simulink model "main_mmp_frac"  (R2024a)
settings: Solver=VariableStepAuto  StartTime=0.0  StopTime=Tsim  FixedStep=simStepSize  RelTol=1e-3
undefined symbols (not defined in the file): A_amp, B_para, f_hz, ForceDist, L_t, mmp_fir_coeff, mmp_iir_coeff, p_off, Ps_sys, Pz_sys, Qcvx_sim, SensorNoise, T_cs, T_fs, T_ss
libraries: cstblocks x2
settings Model: Creator=tomli  LastModifiedBy=tpjch
settings RTWCC: GPUComputeCapability=3.5

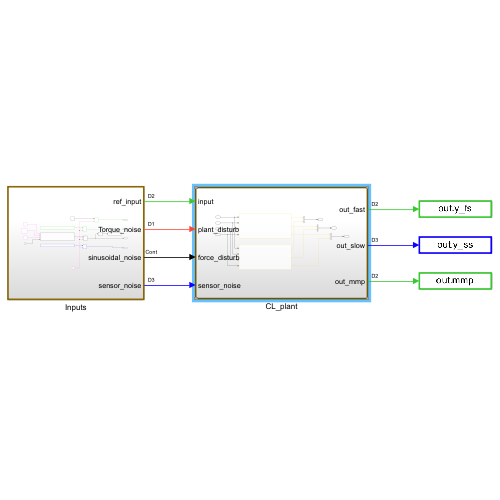
[thumbnail: Simulink's stored preview of the top-level diagram]
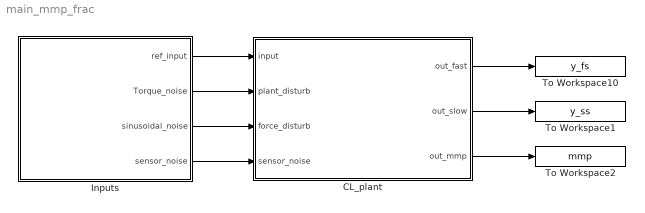
== system main_mmp_frac ==
  CL_plant : Subsystem
  Inputs : Subsystem
  To Workspace1 : ToWorkspace  VariableName=y_ss  SaveFormat=Structure With Time  SampleTime=-1
  To Workspace10 : ToWorkspace  VariableName=y_fs  SaveFormat=Structure With Time  SampleTime=-1
  To Workspace2 : ToWorkspace  VariableName=mmp  SaveFormat=Structure With Time  SampleTime=-1
  wires:
  Inputs/1(ref_input) -> CL_plant/1(input)
  Inputs/2(Torque_noise) -> CL_plant/2(plant_disturb)
  Inputs/3(sinusoidal_noise) -> CL_plant/3(force_disturb)
  Inputs/4(sensor_noise) -> CL_plant/4(sensor_noise)
  CL_plant/1(out_fast) -> To Workspace10/1
  CL_plant/2(out_slow) -> To Workspace1/1
  CL_plant/3(out_mmp) -> To Workspace2/1

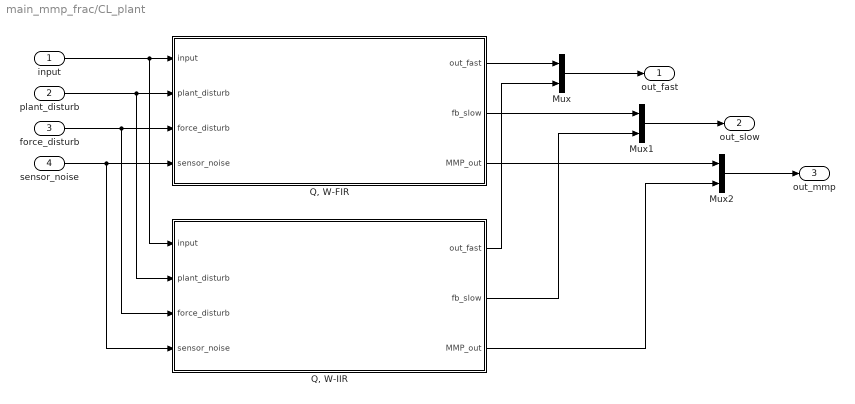
== system main_mmp_frac/CL_plant ==
  input : Inport
  plant_disturb : Inport  Port=2
  force_disturb : Inport  Port=3
  sensor_noise : Inport  Port=4
  Mux : Mux  Inputs=2
  Mux1 : Mux  Inputs=2
  Mux2 : Mux  Inputs=2
  "Q, W-FIR" : Subsystem
  "Q, W-IIR" : Subsystem
  out_fast : Outport
  out_slow : Outport  Port=2
  out_mmp : Outport  Port=3
  wires:
  sensor_noise/1 -> "Q, W-IIR"/4(sensor_noise), "Q, W-FIR"/4(sensor_noise)
  "Q, W-FIR"/2(fb_slow) -> Mux1/1
  Mux1/1 -> out_slow/1
  "Q, W-IIR"/1(out_fast) -> Mux/2
  plant_disturb/1 -> "Q, W-IIR"/2(plant_disturb), "Q, W-FIR"/2(plant_disturb)
  force_disturb/1 -> "Q, W-IIR"/3(force_disturb), "Q, W-FIR"/3(force_disturb)
  "Q, W-FIR"/1(out_fast) -> Mux/1
  input/1 -> "Q, W-IIR"/1(input), "Q, W-FIR"/1(input)
  "Q, W-FIR"/3(MMP_out) -> Mux2/1
  Mux/1 -> out_fast/1
  Mux2/1 -> out_mmp/1
  "Q, W-IIR"/3(MMP_out) -> Mux2/2
  "Q, W-IIR"/2(fb_slow) -> Mux1/2

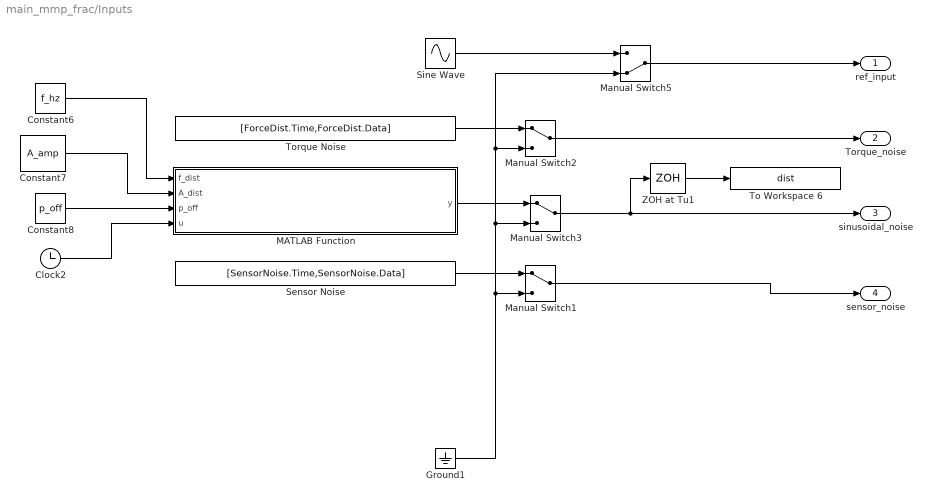
== system main_mmp_frac/Inputs ==
  Clock2 : Clock
  Constant6 : Constant  Value=f_hz
  Constant7 : Constant  Value=A_amp
  Constant8 : Constant  Value=p_off
  Ground1 : Ground
  MATLAB Function : MATLAB Function  TreatAsAtomicUnit=on
  Manual Switch1 : ManualSwitch
  Manual Switch2 : ManualSwitch
  Manual Switch3 : ManualSwitch
  Manual Switch5 : ManualSwitch  CurrentSetting=0
  Sensor Noise : FromWorkspace  VariableName=[SensorNoise.Time,SensorNoise.Data]  SampleTime=SensorNoise.Ts  Interpolate=off  ZeroCross=off  OutputAfterFinalValue=Setting to zero
  Sine Wave : Sin  SampleTime=T_fs
  To Workspace 6 : ToWorkspace  VariableName=dist  SaveFormat=Structure With Time  SampleTime=T_fs
      settings: MaxDataPoints=Inf
  Torque Noise : FromWorkspace  VariableName=[ForceDist.Time,ForceDist.Data]  SampleTime=ForceDist.Ts  Interpolate=off  ZeroCross=off  OutputAfterFinalValue=Setting to zero
  ZOH at Tu1 : ZeroOrderHold  SampleTime=T_fs
  ref_input : Outport
  Torque_noise : Outport  Port=2
  sinusoidal_noise : Outport  Port=3
  sensor_noise : Outport  Port=4
  wires:
  Torque Noise/1 -> Manual Switch2/1
  Constant7/1 -> MATLAB Function/2(A_dist)
  Manual Switch1/1 -> sensor_noise/1
  Constant8/1 -> MATLAB Function/3(p_off)
  MATLAB Function/1(y) -> Manual Switch3/1
  Clock2/1 -> MATLAB Function/4(u)
  Constant6/1 -> MATLAB Function/1(f_dist)
  ZOH at Tu1/1 -> To Workspace 6/1
  Manual Switch3/1 -> sinusoidal_noise/1, ZOH at Tu1/1
  Sensor Noise/1 -> Manual Switch1/1
  Manual Switch2/1 -> Torque_noise/1
  Manual Switch5/1 -> ref_input/1
  Sine Wave/1 -> Manual Switch5/1
  Ground1/1 -> Manual Switch5/2, Manual Switch2/2, Manual Switch3/2, Manual Switch1/2

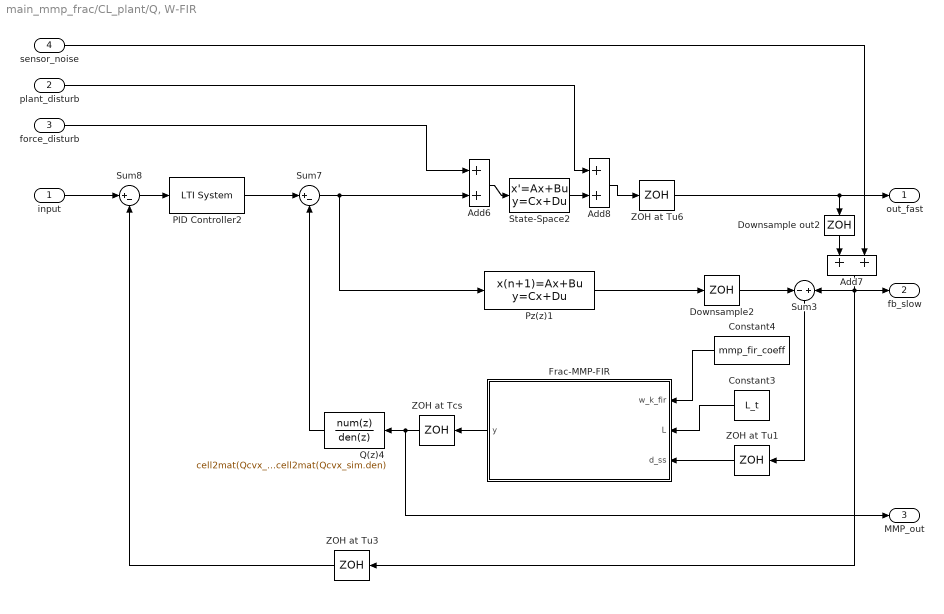
== system main_mmp_frac/CL_plant/Q, W-FIR ==
  input : Inport
  plant_disturb : Inport  Port=2
  force_disturb : Inport  Port=3
  sensor_noise : Inport  Port=4
  Add6 : Sum
  Add7 : Sum
  Add8 : Sum
  Constant3 : Constant  Value=L_t
  Constant4 : Constant  Value=mmp_fir_coeff
  Downsample out2 : ZeroOrderHold  SampleTime=T_ss
  Downsample2 : ZeroOrderHold  SampleTime=T_ss
  Frac-MMP-FIR : Subsystem
  PID Controller2 : cstblocks/LTI System  sys=Cz  IC=[]  PadeOrder=0
  Pz(z)1 : DiscreteStateSpace  A=Pz_sys.A  B=Pz_sys.B  C=Pz_sys.C  D=Pz_sys.D  SampleTime=T_fs
  Q(z)4 : DiscreteTransferFcn  Numerator=cell2mat(Qcvx_sim.num)  Denominator=cell2mat(Qcvx_sim.den)
  State-Space2 : StateSpace  A=Ps_sys.A  B=Ps_sys.B  C=Ps_sys.C  D=Ps_sys.D  InitialCondition=0
  Sum3 : Sum  Inputs=-|+
  Sum7 : Sum  Inputs=|+-
  Sum8 : Sum  Inputs=|+-
  ZOH at Tcs : ZeroOrderHold  SampleTime=T_fs
  ZOH at Tu1 : ZeroOrderHold  SampleTime=T_cs
  ZOH at Tu3 : ZeroOrderHold  SampleTime=T_fs
  ZOH at Tu6 : ZeroOrderHold  SampleTime=T_fs
  out_fast : Outport
  fb_slow : Outport  Port=2
  MMP_out : Outport  Port=3
  wires:
  Q(z)4/1 -> Sum7/2
  ZOH at Tu1/1 -> Frac-MMP-FIR/3(d_ss)
  Frac-MMP-FIR/1(y) -> ZOH at Tcs/1
  Constant4/1 -> Frac-MMP-FIR/1(w_k_fir)
  Constant3/1 -> Frac-MMP-FIR/2(L)
  Sum3/1 -> ZOH at Tu1/1
  Downsample2/1 -> Sum3/1
  ZOH at Tcs/1 -> Q(z)4/1, MMP_out/1
  force_disturb/1 -> Add6/1
  Add6/1 -> State-Space2/1
  ZOH at Tu6/1 -> out_fast/1, Downsample out2/1
  Add8/1 -> ZOH at Tu6/1
  plant_disturb/1 -> Add8/1
  Downsample out2/1 -> Add7/1
  Pz(z)1/1 -> Downsample2/1
  State-Space2/1 -> Add8/2
  ZOH at Tu3/1 -> Sum8/2
  Sum7/1 -> Add6/2, Pz(z)1/1
  sensor_noise/1 -> Add7/2
  Sum8/1 -> PID Controller2/1
  input/1 -> Sum8/1
  PID Controller2/1 -> Sum7/1
  Add7/1 -> ZOH at Tu3/1, fb_slow/1, Sum3/2

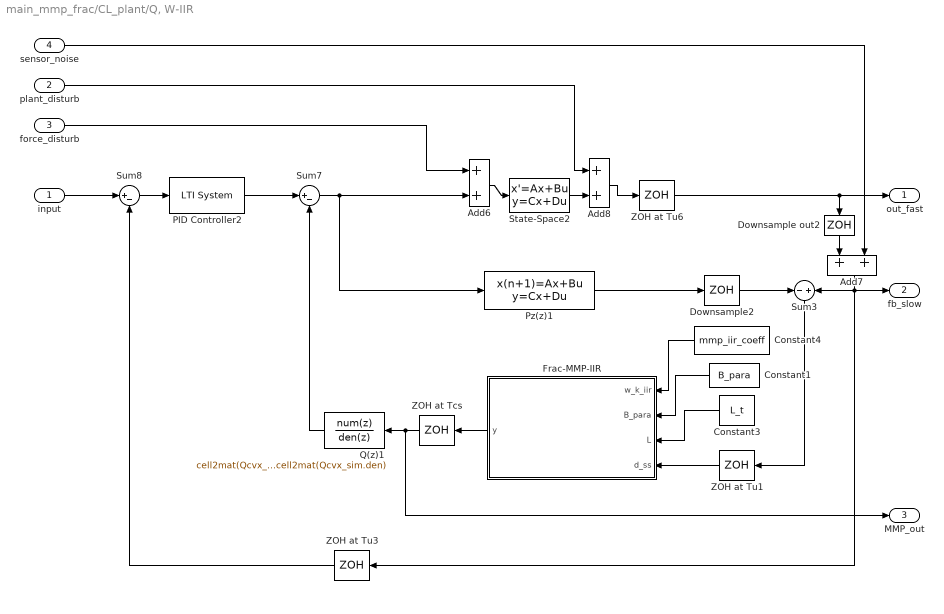
== system main_mmp_frac/CL_plant/Q, W-IIR ==
  input : Inport
  plant_disturb : Inport  Port=2
  force_disturb : Inport  Port=3
  sensor_noise : Inport  Port=4
  Add6 : Sum
  Add7 : Sum
  Add8 : Sum
  Constant1 : Constant  Value=B_para
  Constant3 : Constant  Value=L_t
  Constant4 : Constant  Value=mmp_iir_coeff
  Downsample out2 : ZeroOrderHold  SampleTime=T_ss
  Downsample2 : ZeroOrderHold  SampleTime=T_ss
  Frac-MMP-IIR : Subsystem
  PID Controller2 : cstblocks/LTI System  sys=Cz  IC=[]  PadeOrder=0
  Pz(z)1 : DiscreteStateSpace  A=Pz_sys.A  B=Pz_sys.B  C=Pz_sys.C  D=Pz_sys.D  SampleTime=T_fs
  Q(z)1 : DiscreteTransferFcn  Numerator=cell2mat(Qcvx_sim.num)  Denominator=cell2mat(Qcvx_sim.den)
  State-Space2 : StateSpace  A=Ps_sys.A  B=Ps_sys.B  C=Ps_sys.C  D=Ps_sys.D  InitialCondition=0
  Sum3 : Sum  Inputs=-|+
  Sum7 : Sum  Inputs=|+-
  Sum8 : Sum  Inputs=|+-
  ZOH at Tcs : ZeroOrderHold  SampleTime=T_fs
  ZOH at Tu1 : ZeroOrderHold  SampleTime=T_cs
  ZOH at Tu3 : ZeroOrderHold  SampleTime=T_fs
  ZOH at Tu6 : ZeroOrderHold  SampleTime=T_fs
  out_fast : Outport
  fb_slow : Outport  Port=2
  MMP_out : Outport  Port=3
  wires:
  Add7/1 -> ZOH at Tu3/1, fb_slow/1, Sum3/2
  Sum7/1 -> Add6/2, Pz(z)1/1
  Pz(z)1/1 -> Downsample2/1
  sensor_noise/1 -> Add7/2
  Downsample out2/1 -> Add7/1
  plant_disturb/1 -> Add8/1
  input/1 -> Sum8/1
  Add8/1 -> ZOH at Tu6/1
  Sum8/1 -> PID Controller2/1
  ZOH at Tu3/1 -> Sum8/2
  PID Controller2/1 -> Sum7/1
  Downsample2/1 -> Sum3/1
  force_disturb/1 -> Add6/1
  ZOH at Tcs/1 -> Q(z)1/1, MMP_out/1
  Add6/1 -> State-Space2/1
  Sum3/1 -> ZOH at Tu1/1
  Constant1/1 -> Frac-MMP-IIR/2(B_para)
  Q(z)1/1 -> Sum7/2
  Constant3/1 -> Frac-MMP-IIR/3(L)
  State-Space2/1 -> Add8/2
  Constant4/1 -> Frac-MMP-IIR/1(w_k_iir)
  ZOH at Tu6/1 -> out_fast/1, Downsample out2/1
  ZOH at Tu1/1 -> Frac-MMP-IIR/4(d_ss)
  Frac-MMP-IIR/1(y) -> ZOH at Tcs/1

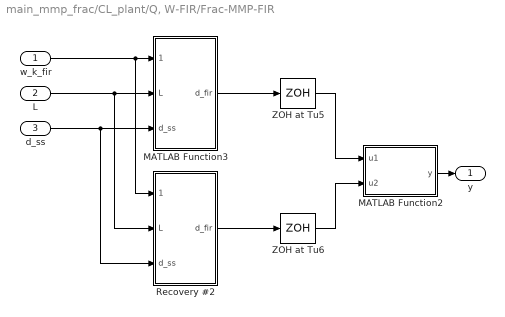
== system main_mmp_frac/CL_plant/Q, W-FIR/Frac-MMP-FIR ==
  w_k_fir : Inport
  L : Inport  Port=2
  d_ss : Inport  Port=3
  MATLAB Function2 : MATLAB Function  TreatAsAtomicUnit=on
  MATLAB Function3 : MATLAB Function  TreatAsAtomicUnit=on  SystemSampleTime=T_cs
  Recovery #2 : MATLAB Function  TreatAsAtomicUnit=on  SystemSampleTime=T_cs
  ZOH at Tu5 : ZeroOrderHold  SampleTime=T_cs
  ZOH at Tu6 : ZeroOrderHold  SampleTime=T_cs
  y : Outport
  wires:
  MATLAB Function2/1(y) -> y/1
  L/1 -> Recovery #2/2(L), MATLAB Function3/2(L)
  w_k_fir/1 -> Recovery #2/1(w_k_fir), MATLAB Function3/1(w_k_fir)
  ZOH at Tu5/1 -> MATLAB Function2/1(u1)
  MATLAB Function3/1(d_fir) -> ZOH at Tu5/1
  Recovery #2/1(d_fir) -> ZOH at Tu6/1
  ZOH at Tu6/1 -> MATLAB Function2/2(u2)
  d_ss/1 -> Recovery #2/3(d_ss), MATLAB Function3/3(d_ss)

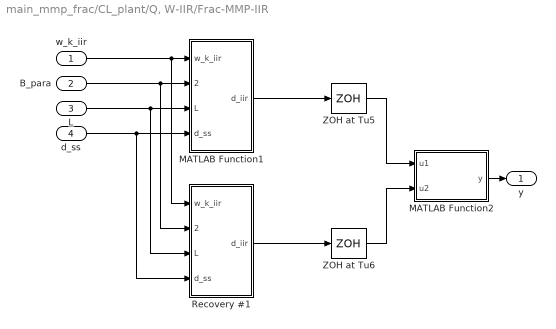
== system main_mmp_frac/CL_plant/Q, W-IIR/Frac-MMP-IIR ==
  w_k_iir : Inport
  B_para : Inport  Port=2
  L : Inport  Port=3
  d_ss : Inport  Port=4
  MATLAB Function1 : MATLAB Function  TreatAsAtomicUnit=on  SystemSampleTime=T_cs
  MATLAB Function2 : MATLAB Function  TreatAsAtomicUnit=on
  Recovery #1 : MATLAB Function  TreatAsAtomicUnit=on  SystemSampleTime=T_cs
  ZOH at Tu5 : ZeroOrderHold  SampleTime=T_cs
  ZOH at Tu6 : ZeroOrderHold  SampleTime=T_cs
  y : Outport
  wires:
  MATLAB Function2/1(y) -> y/1
  L/1 -> Recovery #1/3(L), MATLAB Function1/3(L)
  w_k_iir/1 -> Recovery #1/1(w_k_iir), MATLAB Function1/1(w_k_iir)
  ZOH at Tu5/1 -> MATLAB Function2/1(u1)
  MATLAB Function1/1(d_iir) -> ZOH at Tu5/1
  Recovery #1/1(d_iir) -> ZOH at Tu6/1
  ZOH at Tu6/1 -> MATLAB Function2/2(u2)
  B_para/1 -> Recovery #1/2(B_para), MATLAB Function1/2(B_para)
  d_ss/1 -> Recovery #1/4(d_ss), MATLAB Function1/4(d_ss)

== matlab function main_mmp_frac/Inputs/MATLAB Function ==
  data: f_dist input; A_dist input; p_off input; u input; y output
function y = fcn(f_dist,A_dist,p_off,u)
y = zeros(1,length(u));
for i = 1:length(f_dist)
y = y + A_dist(i)*sin(2*pi*f_dist(i)*u+p_off(i));
end

== matlab function main_mmp_frac/CL_plant/Q, W-IIR/Frac-MMP-IIR/Recovery #1 ==
  settings: updateMethod=DISCRETE
  data: w_k_iir input; B_para input; L input; d_ss input; d_iir output
function d_iir  = fcn(w_k_iir, B_para, L, d_ss)
    % Keeps data of variables
    persistent  n_w phi n_cs n_ss d_buff d_fs_iir max_buffer_size buffer_indices N_L D_L
    % Assigning initial values   
    if isempty(n_w)
        n_w = size(w_k_iir,1); % n_w = 2m disturbances (index starts at 0,1,...,2m-1)
        phi = zeros(1, n_w, 'like', d_ss); % Preallocate phi using the same type as d_ss
        [N_L, D_L] = rat(L);
        n_cs = -N_L; % offset to be one slow sample behind, rate at T_fs/D_L
        n_ss = 0; % Slow sampling count
        d_fs_iir = 0;
        buffer_indices = 2:N_L:((n_w-1) * N_L + 2);
        max_buffer_size = (n_w * N_L + 1);
        d_buff = zeros(1, max_buffer_size, 'like', d_ss);
    end
    
    % Increment fast sampling count
    n_cs = n_cs + 1;
    k = mod(n_cs-1,2*N_L); % check if on intersample
    % Update slow sampling count when k == 0
    if k == 0
        n_ss = n_ss + 1; % Number of slow samples
    end

    % Case 1: n_ss < n_w (not enough data points for FIR)
    if n_ss < n_w
        if k == 0 % Fast and slow align
            phi = [d_ss, phi(1:end-1)]; % Shift and update phi
            d_iir = d_ss;
            d_buff = [d_iir, d_buff(1:end-1)];
        else % Not enough data for intersample estimation
            d_iir = 0;
            d_buff = [d_iir, d_buff(1:end-1)];
        end
    % Case 2: n_ss >= n_w (enough data points for FIR)
    elseif n_ss >= n_w && n_ss < (n_w + 1)
        if k == 0 
            phi = [d_ss, phi(1:end-1)];
            d_iir = d_ss;
            d_buff = [d_iir, d_buff(1:end-1)];
        elseif k ~= 0 && mod(k,2) == 0 % FIR reconstruction
            d_iir = 0;
            d_buff = [d_iir, d_buff(1:end-1)];
        else k ~= 0 && mod(k+1,2) == 0;
            d_iir = 0;
        end
    % Case 3: n_w >= n_w+1, IIR reconstruction
    else
        if k == 0
            phi = [d_ss, phi(1:end-1)];
            d_iir = d_ss;
            d_buff = [d_iir, d_buff(1:end-1)];
        elseif k ~= 0 && mod(k,2) == 0
            d_temp = flip(d_buff);
            d_iir = phi * w_k_iir(:,k/D_L) - ...
                    d_temp(buffer_indices) * flip(B_para(2:end));
            d_buff = [d_iir, d_buff(1:end-1)];
        else k ~= 0 && mod(k+1,2) == 0;
            d_iir = d_fs_iir;
        end
    end
end

== matlab function main_mmp_frac/CL_plant/Q, W-IIR/Frac-MMP-IIR/MATLAB Function1 ==
  settings: updateMethod=DISCRETE
  data: w_k_iir input; B_para input; L input; d_ss input; d_iir output
function d_iir  = fcn(w_k_iir, B_para, L, d_ss)
    % Keeps data of variables
    persistent  n_w phi n_cs n_ss d_buff d_fs_iir max_buffer_size buffer_indices N_L D_L
    % Assigning initial values   
    if isempty(n_w)
        n_w = size(w_k_iir,1); % n_w = 2m disturbances (index starts at 0,1,...,2m-1)
        phi = zeros(1, n_w, 'like', d_ss); % Preallocate phi using the same type as d_ss
        n_cs = 0; % combined sampling count, rate at T_fs/N_L
        n_ss = 0; % Slow sampling count
        d_fs_iir = 0;
        [N_L, D_L] = rat(L);
        buffer_indices = 2:N_L:((n_w-1) * N_L + 2);
        max_buffer_size = (n_w * N_L + 1);
        d_buff = zeros(1, max_buffer_size, 'like', d_ss);
    end
    
    % Increment fast sampling count
    n_cs = n_cs + 1;
    k = mod(n_cs-1,2*N_L); % check if on intersample
    % Update slow sampling count when k == 0
    if k == 0
        n_ss = n_ss + 1; % Number of slow samples
    end

    % Case 1: n_ss < n_w (not enough data points for FIR)
    if n_ss < n_w
        if k == 0 % Fast and slow align
            phi = [d_ss, phi(1:end-1)]; % Shift and update phi
            d_iir = d_ss;
            d_buff = [d_iir, d_buff(1:end-1)];
        else % Not enough data for intersample estimation
            d_iir = 0;
            d_buff = [d_iir, d_buff(1:end-1)];
        end
    % Case 2: n_ss >= n_w (enough data points for FIR)
    elseif n_ss >= n_w && n_ss < (n_w + 1)
        if k == 0 
            phi = [d_ss, phi(1:end-1)];
            d_iir = d_ss;
            d_buff = [d_iir, d_buff(1:end-1)];
        elseif k ~= 0 && mod(k,2) == 0 % FIR reconstruction
            d_iir = 0;
            d_buff = [d_iir, d_buff(1:end-1)];
        else k ~= 0 && mod(k+1,2) == 0;
            d_iir = 0;
        end
    % Case 3: n_w >= n_w+1, IIR reconstruction
    else
        if k == 0
            phi = [d_ss, phi(1:end-1)];
            d_iir = d_ss;
            d_buff = [d_iir, d_buff(1:end-1)];
        elseif k ~= 0 && mod(k,2) == 0
            d_temp = flip(d_buff);
            d_iir = phi * w_k_iir(:,k/D_L) - ...
                    d_temp(buffer_indices) * flip(B_para(2:end));
            d_fs_iir = d_iir;
            d_buff = [d_iir, d_buff(1:end-1)];
        else k ~= 0 && mod(k+1,2) == 0;
            d_iir = d_fs_iir;
        end
    end
    % update buffer
end

== matlab function main_mmp_frac/CL_plant/Q, W-IIR/Frac-MMP-IIR/MATLAB Function2 ==
  data: u1 input; y output; u2 input
function y = summation(u1,u2)

persistent k

if isempty(k)
    k = uint32(0);
end

if mod(k,2) == 0
    y = u1;
else
    y = u2;
end

k = k + 1;

== matlab function main_mmp_frac/CL_plant/Q, W-FIR/Frac-MMP-FIR/MATLAB Function2 ==
  data: u1 input; y output; u2 input
function y = summation(u1,u2)

persistent k

if isempty(k)
    k = uint32(0);
end

if mod(k,2) == 0
    y = u1;
else
    y = u2;
end

k = k + 1;

== matlab function main_mmp_frac/CL_plant/Q, W-FIR/Frac-MMP-FIR/MATLAB Function3 ==
  settings: updateMethod=DISCRETE
  data: w_k_fir input; L input; d_ss input; d_fir output size=1
function d_fir  = fcn(w_k_fir, L, d_ss)
    % Keeps data of variables
    persistent  n_w phi n_cs n_ss d_fs_fir D_L N_L
    % Assigning initial values   
    if isempty(n_w)
        n_w = size(w_k_fir,1); % n_w = 2m disturbances (index starts at 0,1,...,2m-1)
        phi = zeros(1, n_w, 'like', d_ss); % Preallocate phi using the same type as d_ss
        n_cs = 0; % combined sampling count, rate at T_fs/N_L
        n_ss = 0; % Slow sampling count
        d_fs_fir = 0; % store previous value for the estimate
        [N_L, D_L] = rat(L);
    end
    
    % Increment fast sampling count
    n_cs = n_cs + 1;
    k = mod(n_cs-1,2*N_L); % check if on intersample
    % Update slow sampling count when k == 0
    if k == 0
        n_ss = n_ss + 1; % Number of slow samples
    end

    % Case 1: n_ss < n_w (not enough data points for FIR)
    if n_ss < n_w
        if k == 0 % Fast and slow align
            phi = [d_ss, phi(1:end-1)]; % Shift and update phi
            d_fir = d_ss;
        else % Not enough data for intersample estimation
            d_fir = 0;
        end
    % Case 2: n_ss >= n_w (enough data points for FIR)
    else
        if k == 0 
            phi = [d_ss, phi(1:end-1)];
            d_fir = d_ss;
        elseif k ~= 0 && mod(k,2) == 0 % FIR reconstruction
            d_fir = phi * w_k_fir(:, k/D_L); 
            d_fs_fir = d_fir;
        else k ~= 0 && mod(k+1,2) == 0;
            d_fir = d_fs_fir;
        end
    % update buffer
    end

== matlab function main_mmp_frac/CL_plant/Q, W-FIR/Frac-MMP-FIR/Recovery #2 ==
  settings: updateMethod=DISCRETE
  data: w_k_fir input; L input; d_ss input; d_fir output size=1
function d_fir = fcn(w_k_fir, L, d_ss)
    % Keeps data of variables
    persistent  n_w phi n_cs n_ss d_fs_fir N_L D_L
    % Assigning initial values   
    if isempty(n_w)
        n_w = size(w_k_fir,1); % n_w = 2m disturbances (index starts at 0,1,...,2m-1)
        phi = zeros(1, n_w, 'like', d_ss); % Preallocate phi using the same type as d_ss
        [N_L, D_L] = rat(L);
        n_cs = -N_L; % offset to be one slow sample behind, rate at T_fs/D_L
        n_ss = 0; % Slow sampling count
        d_fs_fir = 0; % store previous value for the estimate
    end
    
    % Increment fast sampling count
    n_cs = n_cs + 1;
    k = mod(n_cs-1,2*N_L); % check if on intersample
    % Update slow sampling count when k == 0
    if k == 0
        n_ss = n_ss + 1; % Number of slow samples
    end

    % Case 1: n_ss < n_w (not enough data points for FIR)
    if n_ss < n_w
        if k == 0 % Fast and slow align
            phi = [d_ss, phi(1:end-1)]; % Shift and update phi
            d_fir = d_ss;
        else % Not enough data for intersample estimation
            d_fir = 0;
        end
    % Case 2: n_ss >= n_w (enough data points for FIR)
    else
        if k == 0 
            phi = [d_ss, phi(1:end-1)];
            d_fir = d_ss;
        elseif k ~= 0 && mod(k,2) == 0 % FIR reconstruction
            d_fir = phi * w_k_fir(:, k/D_L); 
            d_fs_fir = d_fir;
        else k ~= 0 && mod(k+1,2) == 0;
            d_fir = d_fs_fir;
        end
    end
